simulink model "lyapunovFinal"  (R2023b)
settings: Solver=VariableStepAuto  StartTime=0.0  StopTime=200  RelTol=1e-3
values from neighbouring files (symbols this model uses):
  Irw = (5.7e-5)*eye(3)    [initialsSpaceCraft.m]
  Jt = [0.185 0 0;0 0.144 0;0 0 0.061]    [initialsSpaceCraft.m]
  K = 2*eye(3)    [initialsSpaceCraft.m]
  omega = zeros(3,1)    [initialsSpaceCraft.m]
  omegades = zeros(3,1)    [initialsSpaceCraft.m]
  omegadotdes = zeros(3,1)    [initialsSpaceCraft.m]
  Q = [0;0;0;1]    [initialsSpaceCraft.m]
  RWvel = 0.*ones(3,1)    [initialsSpaceCraft.m]
  Td = [7.47573281216648e-23 ... (first row only)    [initialsSpaceCraft.m]
settings Model: Creator=Egraweb  LastModifiedBy=s.sh
settings OptimizationCC: ReuseModelBlockBuffer=off

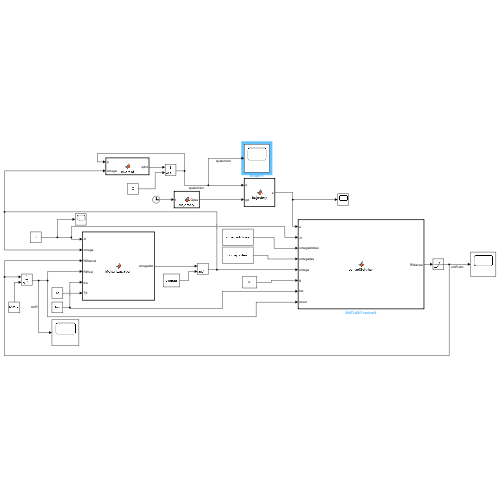
[thumbnail: Simulink's stored preview of the top-level diagram]
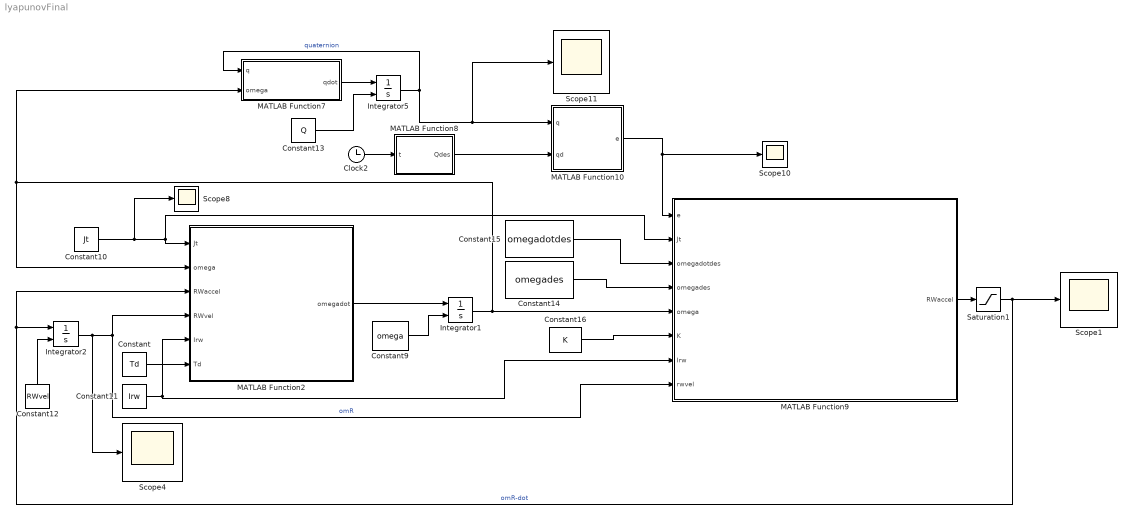
== system lyapunovFinal ==
  Clock2 : Clock
  Constant : Constant  Value=Td
  Constant10 : Constant  Value=Jt
  Constant11 : Constant  Value=Irw
  Constant12 : Constant  Value=RWvel
  Constant13 : Constant  Value=Q
  Constant14 : Constant  Value=omegades
  Constant15 : Constant  Value=omegadotdes
  Constant16 : Constant  Value=K
  Constant9 : Constant  Value=omega
  Integrator1 : Integrator  InitialConditionSource=external
  Integrator2 : Integrator  InitialConditionSource=external
  Integrator5 : Integrator  InitialConditionSource=external
  MATLAB Function10 : MATLAB Function  TreatAsAtomicUnit=on
  MATLAB Function2 : MATLAB Function  TreatAsAtomicUnit=on
  MATLAB Function7 : MATLAB Function  TreatAsAtomicUnit=on
  MATLAB Function8 : MATLAB Function  TreatAsAtomicUnit=on
  MATLAB Function9 : MATLAB Function  TreatAsAtomicUnit=on
  Saturation1 : Saturate  UpperLimit=176  LowerLimit=-176  LinearizeAsGain=off  RndMeth=Ceiling
  Scope{1,4,8,10..11} (5 alike) : Scope
  wires:
  Constant12/1 -> Integrator2/2
  Constant10/1 -> MATLAB Function9/2(Jt), MATLAB Function2/1(Jt), Scope8/1
  MATLAB Function8/1(Qdes) -> MATLAB Function10/2(qd)
  Integrator5/1 -> MATLAB Function7/1(q), Scope11/1, MATLAB Function10/1(q)  "quaternion"
  MATLAB Function2/1(omegadot) -> Integrator1/1
  Constant9/1 -> Integrator1/2
  Integrator2/1 -> Scope4/1, MATLAB Function9/8(rwvel), MATLAB Function2/4(RWvel)  "omR"
  Clock2/1 -> MATLAB Function8/1(t)
  MATLAB Function10/1(e) -> MATLAB Function9/1(e), Scope10/1
  Constant14/1 -> MATLAB Function9/4(omegades)
  MATLAB Function9/1(RWaccel) -> Saturation1/1
  Saturation1/1 -> Integrator2/1, MATLAB Function2/3(RWaccel), Scope1/1  "omR-dot"
  Constant15/1 -> MATLAB Function9/3(omegadotdes)
  Constant13/1 -> Integrator5/2
  MATLAB Function7/1(qdot) -> Integrator5/1
  Constant11/1 -> MATLAB Function2/5(Irw), MATLAB Function9/7(Irw)
  Constant16/1 -> MATLAB Function9/6(K)
  Integrator1/1 -> MATLAB Function9/5(omega), MATLAB Function2/2(omega), MATLAB Function7/2(omega)
  Constant/1 -> MATLAB Function2/6(Td)

== matlab function lyapunovFinal/MATLAB Function10 ==
  data: q input; e output; qd input
function e = trajectory(q,qd)
qd1=qd(1);qd2=qd(2);qd3=qd(3);qd4=qd(4);
qe=[qd4 qd3 -qd2 -qd1;-qd3 qd4 qd1 -qd2;qd2 -qd1 qd4 -qd3;qd1 qd2 qd3 qd4]*q;
e=qe(1:3);

== matlab function lyapunovFinal/MATLAB Function8 ==
  data: t input; Qdes output
function Qdes = trajectory(t)

 Qdes=[1;0;0;0];

== matlab function lyapunovFinal/MATLAB Function2 ==
  data: Jt input; omega input; RWaccel input; RWvel input; omegadot output; Irw input; Td input
function omegadot = MotionEquation(Jt,omega,RWaccel,RWvel,Irw , Td)
alpha=RWaccel;
w=RWvel;
Tc=0;
omegadot=Jt^-1*(Tc+Td-Irw*alpha-omega.*(Jt*omega+Irw*w));

== matlab function lyapunovFinal/MATLAB Function7 ==
  data: q input; qdot output; omega input
function qdot = quatdot(q,omega)
wB1=omega(1);wB2=omega(2);wB3=omega(3);

qdot=0.5*[0 wB3 -wB2 wB1;-wB3 0 wB1 wB2;wB2 -wB1 0 wB3;-wB1 -wB2 -wB3 0]*q;

== matlab function lyapunovFinal/MATLAB Function9 ==
  data: e input; Jt input; omegadotdes input; omegades input; omega input; K input; Irw input; rwvel input; RWaccel output
function RWaccel  = controlSolution(e,Jt,omegadotdes,omegades,omega,K,Irw,rwvel)
w=rwvel;
TB=zeros(3,1);
A=0.5*omega+omegades+w;
omega_e=omega-omegades;
B=-Jt*omegadotdes+e+K*omega_e-omega.*(Jt*omega+Irw*w)+TB;
A1=A(1);A2=A(2);A3=A(3);


RWaccel=Irw^-1*B;
